simulink model "STDiscovery2016a"  (R2017b)
settings: Solver=FixedStepAuto  StartTime=0.0  StopTime=10  FixedStep=Abtastzeit  RelTol=1e-3
PreLoadFcn:
  | waijung.modelPreload; % Required for working with Waijung Blockset. Do not remove.
model workspace (MAT data in the model file):
  Abtastzeit = 0.01
  Servo_IN_min = 0.894
  SimulationDutyCycle = 27
undefined symbols (not defined in the file): HSEOSC, Link, LQFP176, ST, STM32F417IG
libraries: stm32f4_io_lib x15, simulink x10, simulink_extras x8, stm32f4_adc_lib x7, powerlib_meascontrol x3, stm32f4_device_config_lib x1
(part 5 of 5)

== system STDiscovery2016a/Aktorik/Ansteuerung Servo/Logik  ==
  Fernbedienung Signal : Inport
  Eingriff_Fernbedienung : Inport  Port=2
  Jetson Signal : Inport  Port=3
  "(Einschaltverzögerung) Wartezeit Anhalten " : powerlib_meascontrol/Logic/On Delay  DelayType=On delay  delay=1  ic=1  Ts=0
      settings: SourceProductName=Simscape Power Systems
  Data Type Conversion : DataTypeConversion  OutDataTypeStr=double
  "Erst 1s aktuellen autonomen Lenkeinschlag halten, dann Fernbedienung übernehmen" : Switch  Criteria=u2 > Threshold
  Modus Auswahl : Switch  Criteria=u2 > Threshold
  Output Pin : Outport
  wires:
  Data Type Conversion/1 -> "Erst 1s aktuellen autonomen Lenkeinschlag halten, dann Fernbedienung übernehmen"/1  "manuell"
  Eingriff_Fernbedienung/1 -> "(Einschaltverzögerung) Wartezeit Anhalten "/1, Modus Auswahl/2
  Modus Auswahl/1 -> Output Pin/1  "Ausgang zum servo"
  "Erst 1s aktuellen autonomen Lenkeinschlag halten, dann Fernbedienung übernehmen"/1 -> Modus Auswahl/1  "manuell"
  Jetson Signal/1 -> Modus Auswahl/3, "Erst 1s aktuellen autonomen Lenkeinschlag halten, dann Fernbedienung übernehmen"/3  "autonom"
  "(Einschaltverzögerung) Wartezeit Anhalten "/1 -> "Erst 1s aktuellen autonomen Lenkeinschlag halten, dann Fernbedienung übernehmen"/2
  Fernbedienung Signal/1 -> Data Type Conversion/1

== system STDiscovery2016a/Aktorik/Ansteuerung Servo/Plausibilitäts Check ==
  In1 : Inport
  "Gib Mittelstellung aus, wenn mit Signal etwas nicht Stimmt" : Switch  Criteria=u2 > Threshold
  Logical Operator : Logic  AllPortsSameDT=off  OutDataTypeStr=boolean
  Mittelstellung : Constant  Value=0.001407
  Relational Operator : RelationalOperator  Operator=<  OutDataTypeStr=boolean  RndMeth=Nearest
  Relational Operator1 : RelationalOperator  Operator=>  OutDataTypeStr=boolean  RndMeth=Nearest
  "ok max " : Constant  Value=0.0021
  ok min : Constant  Value=0.0008
  Out1 : Outport
  wires:
  In1/1 -> Relational Operator1/1, Relational Operator/1, "Gib Mittelstellung aus, wenn mit Signal etwas nicht Stimmt"/1
  Logical Operator/1 -> "Gib Mittelstellung aus, wenn mit Signal etwas nicht Stimmt"/2
  "Gib Mittelstellung aus, wenn mit Signal etwas nicht Stimmt"/1 -> Out1/1
  Mittelstellung/1 -> "Gib Mittelstellung aus, wenn mit Signal etwas nicht Stimmt"/3
  Relational Operator1/1 -> Logical Operator/2
  Relational Operator/1 -> Logical Operator/1
  ok min/1 -> Relational Operator1/2
  "ok max "/1 -> Relational Operator/2

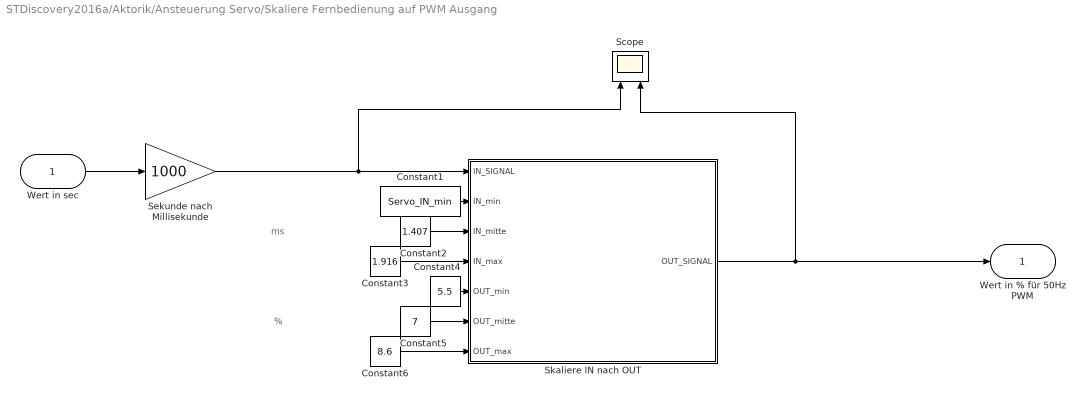
== system STDiscovery2016a/Aktorik/Ansteuerung Servo/Skaliere Fernbedienung auf PWM Ausgang ==
  note: %
  note: ms
  Wert in sec : Inport
  Constant1 : Constant  Value=Servo_IN_min
  Constant2 : Constant  Value=1.407
  Constant3 : Constant  Value=1.916
  Constant4 : Constant  Value=5.5
  Constant5 : Constant  Value=7
  Constant6 : Constant  Value=8.6
  Scope : Scope  NumInputPorts=2
  Sekunde nach Millisekunde : Gain  Gain=1000
  Skaliere lN nach OUT : Subsystem
  Wert in % für 50Hz PWM : Outport
  wires:
  Constant4/1 -> Skaliere lN nach OUT/5(OUT_min)
  Wert in sec/1 -> Sekunde nach Millisekunde/1
  Constant5/1 -> Skaliere lN nach OUT/6(OUT_mitte)
  Skaliere lN nach OUT/1(OUT_SIGNAL) -> Scope/2, Wert in % für 50Hz PWM/1
  Constant3/1 -> Skaliere lN nach OUT/4(IN_max)
  Constant2/1 -> Skaliere lN nach OUT/3(IN_mitte)
  Constant1/1 -> Skaliere lN nach OUT/2(IN_min)
  Constant6/1 -> Skaliere lN nach OUT/7(OUT_max)
  Sekunde nach Millisekunde/1 -> Scope/1, Skaliere lN nach OUT/1(IN_SIGNAL)

== system STDiscovery2016a/Aktorik/Ansteuerung Servo/Skaliere Stellwinkel auf PWM Ausgang ==
  note: %
  note: Stellwinkel
  Stellwinkel : Inport
  Constant1 : Constant  Value=-27
  Constant2 : Constant  Value=0
  Constant3 : Constant  Value=27
  Constant4 : Constant  Value=5.5
  Constant5 : Constant  Value=7
  Constant6 : Constant  Value=8.6
  Skaliere lN nach OUT : Subsystem
  Wert in % für 50Hz PWM : Outport
  wires:
  Constant4/1 -> Skaliere lN nach OUT/5(OUT_min)
  Constant5/1 -> Skaliere lN nach OUT/6(OUT_mitte)
  Skaliere lN nach OUT/1(OUT_SIGNAL) -> Wert in % für 50Hz PWM/1
  Constant3/1 -> Skaliere lN nach OUT/4(IN_max)
  Constant2/1 -> Skaliere lN nach OUT/3(IN_mitte)
  Constant1/1 -> Skaliere lN nach OUT/2(IN_min)
  Constant6/1 -> Skaliere lN nach OUT/7(OUT_max)
  Stellwinkel/1 -> Skaliere lN nach OUT/1(IN_SIGNAL)

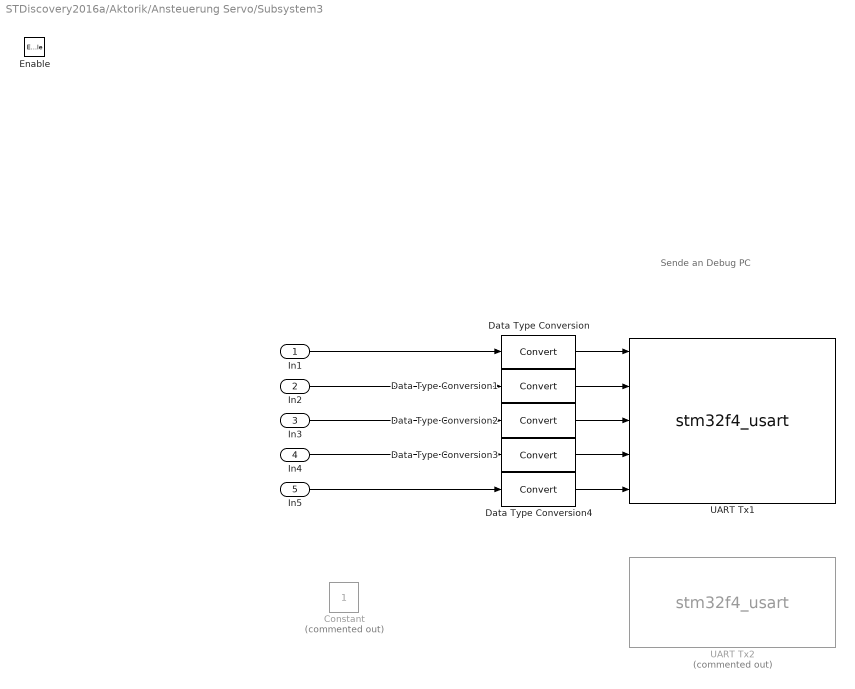
== system STDiscovery2016a/Aktorik/Ansteuerung Servo/Subsystem3 ==
  note: Sende an Debug PC
  In1 : Inport
  In2 : Inport  Port=2
  In3 : Inport  Port=3
  In4 : Inport  Port=4
  In5 : Inport  Port=5
  Enable : EnablePort
  Constant : Constant  Commented=on
  Data Type Conversion{,1..4} (5 alike) : DataTypeConversion
  UART Tx1 : S-Function  Priority=1  FunctionName=stm32f4_usart  Parameters=configuration,uartmodule,transfer,baudrate,inputtype,outputtype,confstr,binheaderarray,binterminatorarray,asciiheader,asciiterminator,bindatalength,packetmode,varname,sampletime,sampletimestr,blockid  SFunctionDeploymentMode=off  EnableBusSupport=off  mask(stm32f4_usart){configuration=Tx, uartmodule=3, baudrate=115200, databits=8, parity=No, stopbit=1, remaptxpin=Not used, remaprxpin=Not used, flowcontrol=None, remapctspin=Not used, remaprtspin=Not used, advanceoptions=off, rxbuffersize=512, txbuffersize=512, transfer=Blocking, packetmode=Ascii, binheader='7E 7E', binterminator='03 03', porttype_double=1, porttype_single=0, porttype_int8=1, porttype_uint8=0, porttype_int16=0, porttype_uint16=0, porttype_int32=0, porttype_uint32=0, asciiformat=' X: %f   ,Y:  %f , Lookahead: %f  , Geschwindigkeit: %f   ,Steuerbits(32):  %f', rx_asciiterminator=CRLF (0x0D 0x0A - "\r\n"), tx_asciiterminator=CRLF (0x0D 0x0A - "\r\n"), storagename=S, varname=, inputtype=[5  1 1 1 1 1], outputtype=[0], binheaderarray=[0], binterminatorarray=[0], bindatalength=0, asciiheader=' X: %f   ,Y:  %f , Lookahead: %f  , Geschwindigkeit: %f   ,Steuerbits(32):  %f\r\n', asciiterminator=[2 13 10], sampletime=0.1, sampletimestr=0.1, blockid=AktorikAnsteuerungServoSubsystem3UARTTx1, confstr=[ "dummy", "0", "*", "*", "0", "*", "*", "0", "*", "*", "0", "*", "*", "1", "4", "3", "1", "4", "1", "512", "512", "1", "3", "115200", "8", "No", "1", "None", "USART3"], lastmodule=1}
      mask prompts: uartmodule "UART Module"; baudrate "Baud rate (bps)"; databits "Data bits"; stopbit "Stop bit"; remaptxpin "Tx Pin"; remaprxpin "Rx Pin"; flowcontrol "Hardware flow control"; remapctspin "HW Flow control, CTS Pin"; remaprtspin "HW Flow control, RTS Pin"; advanceoptions "Advance options"; rxbuffersize "Rx buffer size (bytes)"; txbuffersize "Tx buffer size (bytes)"; packetmode "Packet mode"; binheader "Binary header (example: '7E 7E')"; binterminator "Binary terminator (example: '03 03')"; porttype_double "Number of data port, type DOUBLE"; porttype_single "Number of data port, type SINGLE"; porttype_int8 "Number of data port, type INT8"; porttype_uint8 "Number of data port, type UINT8"; porttype_int16 "Number of data port, type INT16"; porttype_uint16 "Number of data port, type UINT16"; porttype_int32 "Number of data port, type INT32"; porttype_uint32 "Number of data port, type UINT32"; asciiformat "Ascii format"; rx_asciiterminator "End of packet"; tx_asciiterminator "End of packet"; storagename "Buffer"; varname "Var name"; inputtype "Input data type"; outputtype "Output data type"; binheaderarray "Binary header"; binterminatorarray "Binary terminator"; bindatalength "Binary data length"; asciiheader "Ascii header (printf format)"; asciiterminator "Ascii terminator"; sampletime "Sample time (sec)"; sampletimestr "Compiled sample time (sec) in string"; confstr "Configuration string"; lastmodule "Last module selected"
      mask help:
      | Data type for Ascii format
      | %u, %i, %d, %o, %x: uint32
      | %e, %g, %f: single
      | %c: int8
      mask init:
      | stm32f4_usart_callback('init');
      mask Help: web(fullfile(waijungdocroot,'stm32f4_usart_tx.htm'), '-browser')
      mask TypeOptions configuration: Setup | Tx | Rx
      mask Callback configuration: stm32f4_usart_callback('configuration');
      mask TypeOptions uartmodule: 1 | 2 | 3 | 4 | 5 | 6
      mask Callback uartmodule: stm32f4_usart_callback('uartmodule');
      mask Callback baudrate: stm32f4_usart_callback('baudrate');
      mask TypeOptions databits: 8
      mask TypeOptions parity: No | Odd | Even
      mask TypeOptions stopbit: 0.5 | 1 | 1.5 | 2
      mask TypeOptions remaptxpin: Not used | A9 | B6
      mask TypeOptions remaprxpin: Not used | A10 | B7
      mask TypeOptions flowcontrol: None | RTS | CTS | RTS/CTS
      mask Callback flowcontrol: stm32f4_usart_callback('flowcontrol');
      mask TypeOptions remapctspin: Not used | A11
      mask TypeOptions remaprtspin: Not used | A12
      mask Callback advanceoptions: stm32f4_usart_callback('advanceoptions');
      mask TypeOptions rxbuffersize: 16 | 32 | 64 | 128 | 256 | 512 | 1024 | 2048
      mask TypeOptions txbuffersize: 16 | 32 | 64 | 128 | 256 | 512 | 1024 | 2048
      mask TypeOptions transfer: Blocking | Non-Blocking
      mask Callback transfer: stm32f4_usart_callback('transfer');
      mask TypeOptions packetmode: Ascii | Binary | String Buffer
      mask Callback packetmode: stm32f4_usart_callback('packetmode');
      mask Callback binheader: stm32f4_usart_callback('binheader');
      mask Callback binterminator: stm32f4_usart_callback('binterminator');
      mask Callback porttype_double: stm32f4_usart_callback('porttype');
      mask Callback porttype_single: stm32f4_usart_callback('porttype');
      mask Callback porttype_int8: stm32f4_usart_callback('porttype');
      mask Callback porttype_uint8: stm32f4_usart_callback('porttype');
      mask Callback porttype_int16: stm32f4_usart_callback('porttype');
      mask Callback porttype_uint16: stm32f4_usart_callback('porttype');
      mask Callback porttype_int32: stm32f4_usart_callback('porttype');
      mask Callback porttype_uint32: stm32f4_usart_callback('porttype');
      mask Callback asciiformat: stm32f4_usart_callback('asciiformat');
      mask TypeOptions rx_asciiterminator: CR (0x0D - "\r") | LF (0x0A - "\n") | CRLF (0x0D 0x0A - "\r\n")
      mask Callback rx_asciiterminator: stm32f4_usart_callback('rx_asciiterminator');
      mask TypeOptions tx_asciiterminator: CR (0x0D - "\r") | LF (0x0A - "\n") | CRLF (0x0D 0x0A - "\r\n") | None
      mask Callback tx_asciiterminator: stm32f4_usart_callback('tx_asciiterminator');
      mask TypeOptions storagename: <Please insert a storage name> | S
      mask Callback storagename: stm32f4_usart_callback('storagename');
      mask Callback varname: stm32f4_usart_callback('varname');
      mask Callback sampletime: stm32f4_usart_callback('sampletime');
      mask Callback sampletimestr: stm32f4_usart_callback('sampletimestr');
      mask Callback blockid: stm32f4_usart_callback('blockid');
      mask Display: text(0.95, 0.5, 'Module: USART3_Tx\nPacket: Ascii\nTransfer: Blocking\nTs (sec): 0.1','ver','middle','hor','right'); port_label('input', 1,'single'); port_label('input', 2,'single'); port_label('input', 3,'single'); port_label('input', 4,'single'); port_label('input', 5,'single');
  UART Tx2 : S-Function  Priority=1  Commented=on  FunctionName=stm32f4_usart  Parameters=configuration,uartmodule,transfer,baudrate,inputtype,outputtype,confstr,binheaderarray,binterminatorarray,asciiheader,asciiterminator,bindatalength,packetmode,varname,sampletime,sampletimestr,blockid  SFunctionDeploymentMode=off  EnableBusSupport=off  mask(stm32f4_usart){configuration=Tx, uartmodule=1, baudrate=115200, databits=8, parity=No, stopbit=1, remaptxpin=Not used, remaprxpin=Not used, flowcontrol=None, remapctspin=Not used, remaprtspin=Not used, advanceoptions=off, rxbuffersize=512, txbuffersize=512, transfer=Blocking, packetmode=Binary, binheader='', binterminator='', porttype_double=0, porttype_single=1, porttype_int8=0, porttype_uint8=0, porttype_int16=0, porttype_uint16=0, porttype_int32=0, porttype_uint32=0, asciiformat='Lookahead: %f   , X: %f   ,Y:  %f  ,Steuerbits(32):  %f', rx_asciiterminator=CRLF (0x0D 0x0A - "\r\n"), tx_asciiterminator=CRLF (0x0D 0x0A - "\r\n"), storagename=S, varname=, inputtype=[1  1], outputtype=[0], binheaderarray=[0 ], binterminatorarray=[0 ], bindatalength=4, asciiheader='Lookahead: %f   , X: %f   ,Y:  %f  ,Steuerbits(32):  %f\r\n', asciiterminator=[2 13 10], sampletime=0.1, sampletimestr=-1, blockid=AktorikAnsteuerungServoSubsystem3UARTTx2, confstr=[ "dummy", "0", "*", "*", "0", "*", "*", "0", "*", "*", "0", "*", "*", "2", "4", "7", "2", "4", "2", "512", "512", "2", "1", "115200", "8", "No", "1", "None", "USART1"], lastmodule=1}
      mask prompts: uartmodule "UART Module"; baudrate "Baud rate (bps)"; databits "Data bits"; stopbit "Stop bit"; remaptxpin "Tx Pin"; remaprxpin "Rx Pin"; flowcontrol "Hardware flow control"; remapctspin "HW Flow control, CTS Pin"; remaprtspin "HW Flow control, RTS Pin"; advanceoptions "Advance options"; rxbuffersize "Rx buffer size (bytes)"; txbuffersize "Tx buffer size (bytes)"; packetmode "Packet mode"; binheader "Binary header (example: '7E 7E')"; binterminator "Binary terminator (example: '03 03')"; porttype_double "Number of data port, type DOUBLE"; porttype_single "Number of data port, type SINGLE"; porttype_int8 "Number of data port, type INT8"; porttype_uint8 "Number of data port, type UINT8"; porttype_int16 "Number of data port, type INT16"; porttype_uint16 "Number of data port, type UINT16"; porttype_int32 "Number of data port, type INT32"; porttype_uint32 "Number of data port, type UINT32"; asciiformat "Ascii format"; rx_asciiterminator "End of packet"; tx_asciiterminator "End of packet"; storagename "Buffer"; varname "Var name"; inputtype "Input data type"; outputtype "Output data type"; binheaderarray "Binary header"; binterminatorarray "Binary terminator"; bindatalength "Binary data length"; asciiheader "Ascii header (printf format)"; asciiterminator "Ascii terminator"; sampletime "Sample time (sec)"; sampletimestr "Compiled sample time (sec) in string"; confstr "Configuration string"; lastmodule "Last module selected"
      mask help:
      | Data type for Ascii format
      | %u, %i, %d, %o, %x: uint32
      | %e, %g, %f: single
      | %c: int8
      mask init:
      | stm32f4_usart_callback('init');
      mask Help: web(fullfile(waijungdocroot,'stm32f4_usart_tx.htm'), '-browser')
      mask TypeOptions configuration: Setup | Tx | Rx
      mask Callback configuration: stm32f4_usart_callback('configuration');
      mask TypeOptions uartmodule: 1 | 2 | 3 | 4 | 5 | 6
      mask Callback uartmodule: stm32f4_usart_callback('uartmodule');
      mask Callback baudrate: stm32f4_usart_callback('baudrate');
      mask TypeOptions databits: 8
      mask TypeOptions parity: No | Odd | Even
      mask TypeOptions stopbit: 0.5 | 1 | 1.5 | 2
      mask TypeOptions remaptxpin: Not used | A9 | B6
      mask TypeOptions remaprxpin: Not used | A10 | B7
      mask TypeOptions flowcontrol: None | RTS | CTS | RTS/CTS
      mask Callback flowcontrol: stm32f4_usart_callback('flowcontrol');
      mask TypeOptions remapctspin: Not used | A11
      mask TypeOptions remaprtspin: Not used | A12
      mask Callback advanceoptions: stm32f4_usart_callback('advanceoptions');
      mask TypeOptions rxbuffersize: 16 | 32 | 64 | 128 | 256 | 512 | 1024 | 2048
      mask TypeOptions txbuffersize: 16 | 32 | 64 | 128 | 256 | 512 | 1024 | 2048
      mask TypeOptions transfer: Blocking | Non-Blocking
      mask Callback transfer: stm32f4_usart_callback('transfer');
      mask TypeOptions packetmode: Ascii | Binary | String Buffer
      mask Callback packetmode: stm32f4_usart_callback('packetmode');
      mask Callback binheader: stm32f4_usart_callback('binheader');
      mask Callback binterminator: stm32f4_usart_callback('binterminator');
      mask Callback porttype_double: stm32f4_usart_callback('porttype');
      mask Callback porttype_single: stm32f4_usart_callback('porttype');
      mask Callback porttype_int8: stm32f4_usart_callback('porttype');
      mask Callback porttype_uint8: stm32f4_usart_callback('porttype');
      mask Callback porttype_int16: stm32f4_usart_callback('porttype');
      mask Callback porttype_uint16: stm32f4_usart_callback('porttype');
      mask Callback porttype_int32: stm32f4_usart_callback('porttype');
      mask Callback porttype_uint32: stm32f4_usart_callback('porttype');
      mask Callback asciiformat: stm32f4_usart_callback('asciiformat');
      mask TypeOptions rx_asciiterminator: CR (0x0D - "\r") | LF (0x0A - "\n") | CRLF (0x0D 0x0A - "\r\n")
      mask Callback rx_asciiterminator: stm32f4_usart_callback('rx_asciiterminator');
      mask TypeOptions tx_asciiterminator: CR (0x0D - "\r") | LF (0x0A - "\n") | CRLF (0x0D 0x0A - "\r\n") | None
      mask Callback tx_asciiterminator: stm32f4_usart_callback('tx_asciiterminator');
      mask TypeOptions storagename: <Please insert a storage name> | S
      mask Callback storagename: stm32f4_usart_callback('storagename');
      mask Callback varname: stm32f4_usart_callback('varname');
      mask Callback sampletime: stm32f4_usart_callback('sampletime');
      mask Callback sampletimestr: stm32f4_usart_callback('sampletimestr');
      mask Callback blockid: stm32f4_usart_callback('blockid');
      mask Display: text(0.95, 0.5, 'Module: USART1_Tx\nPacket: Binary\nTransfer: Blocking\nTs (sec): -1','ver','middle','hor','right'); port_label('input', 1,'single');
  wires:
  In1/1 -> Data Type Conversion/1
  In2/1 -> Data Type Conversion1/1
  Data Type Conversion/1 -> UART Tx1/1
  Data Type Conversion2/1 -> UART Tx1/3
  Data Type Conversion1/1 -> UART Tx1/2
  In3/1 -> Data Type Conversion2/1
  In4/1 -> Data Type Conversion3/1
  Data Type Conversion3/1 -> UART Tx1/4
  In5/1 -> Data Type Conversion4/1
  Data Type Conversion4/1 -> UART Tx1/5

== system STDiscovery2016a/Aktorik/Ueberwachung ob Eingriff durch Fernbedienung/Motor Überwachung Eingriff durch Fernbedienung? ==
  Dutycycle in % : Inport
  Betrag bilden für negative Abweichunge : Abs
  Ist die Aktuelle Abweichung größer als die Maximal erlaubte? : RelationalOperator  Operator=>  OutDataTypeStr=boolean  RndMeth=Nearest
  Maximale Abweichung : Constant  Value=0.2
  "Mittelwert, in % wenn Fernsteuerung in der Mitte steht" : Constant  Value=7.45
  Subtract : Sum  Inputs=|+-
  Ja/Nein : Outport
  wires:
  "Mittelwert, in % wenn Fernsteuerung in der Mitte steht"/1 -> Subtract/2
  Betrag bilden für negative Abweichunge/1 -> Ist die Aktuelle Abweichung größer als die Maximal erlaubte?/1
  Maximale Abweichung/1 -> Ist die Aktuelle Abweichung größer als die Maximal erlaubte?/2
  Dutycycle in %/1 -> Subtract/1
  Subtract/1 -> Betrag bilden für negative Abweichunge/1
  Ist die Aktuelle Abweichung größer als die Maximal erlaubte?/1 -> Ja/Nein/1

== system STDiscovery2016a/Aktorik/Ueberwachung ob Eingriff durch Fernbedienung/Servo Überwachung Eingriff durch Fernbedienung? ==
  Dutycycle in % : Inport
  Betrag bilden für negative Abweichungen : Abs
  Ist die aktuelle Abweichung größer als die maximal erlaubte? : RelationalOperator  Operator=>  OutDataTypeStr=boolean  RndMeth=Nearest
  Maximale Abweichung : Constant  Value=0.2
  "Mittelwert, in % wenn Fernsteuerung in der Mitte steht" : Constant  Value=7
  Subtract : Sum  Inputs=|+-
  Ja/Nein : Outport
  wires:
  "Mittelwert, in % wenn Fernsteuerung in der Mitte steht"/1 -> Subtract/2
  Betrag bilden für negative Abweichungen/1 -> Ist die aktuelle Abweichung größer als die maximal erlaubte?/1
  Maximale Abweichung/1 -> Ist die aktuelle Abweichung größer als die maximal erlaubte?/2
  Dutycycle in %/1 -> Subtract/1
  Subtract/1 -> Betrag bilden für negative Abweichungen/1
  Ist die aktuelle Abweichung größer als die maximal erlaubte?/1 -> Ja/Nein/1

== system STDiscovery2016a/Debug/Subsystem/Safety 2.5 |<--->|12.5 ==
  In1 : Inport
  Constant : Constant  Value=2.5
  Constant1 : Constant  Value=12.5
  Data Type Conversion : DataTypeConversion
  Data Type Conversion1 : DataTypeConversion
  Switch : Switch  Criteria=u2 > Threshold  Threshold=2.5
  Switch1 : Switch  Criteria=u2 > Threshold  Threshold=12.5
  Out1 : Outport
  wires:
  Switch/1 -> Switch1/3, Switch1/2
  In1/1 -> Switch/1, Switch/2
  Switch1/1 -> Out1/1
  Constant/1 -> Data Type Conversion/1
  Constant1/1 -> Data Type Conversion1/1
  Data Type Conversion1/1 -> Switch1/1
  Data Type Conversion/1 -> Switch/3

== system STDiscovery2016a/Debug/Subsystem1/Safety 2.5 |<--->|12.5 ==
  In1 : Inport
  Constant : Constant  Value=2.5
  Constant1 : Constant  Value=12.5
  Data Type Conversion : DataTypeConversion
  Data Type Conversion1 : DataTypeConversion
  Switch : Switch  Criteria=u2 > Threshold  Threshold=2.5
  Switch1 : Switch  Criteria=u2 > Threshold  Threshold=12.5
  Out1 : Outport
  wires:
  Switch/1 -> Switch1/3, Switch1/2
  In1/1 -> Switch/1, Switch/2
  Switch1/1 -> Out1/1
  Constant/1 -> Data Type Conversion/1
  Constant1/1 -> Data Type Conversion1/1
  Data Type Conversion1/1 -> Switch1/1
  Data Type Conversion/1 -> Switch/3

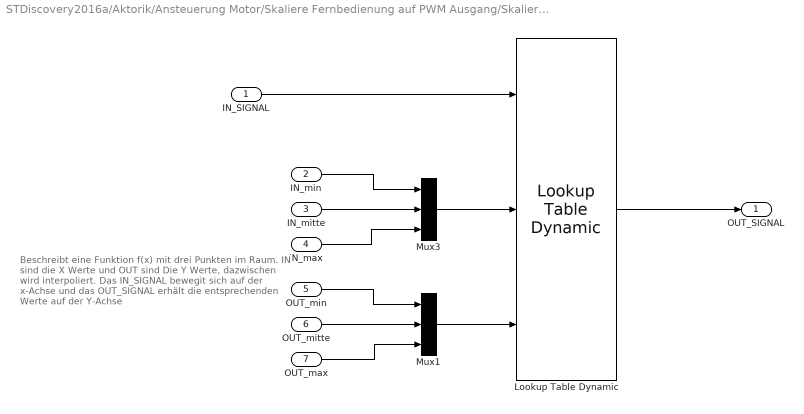
== system STDiscovery2016a/Aktorik/Ansteuerung Motor/Skaliere Fernbedienung auf PWM Ausgang/Skaliere lN nach OUT ==
  note: Beschreibt eine Funktion f(x) mit drei Punkten im Raum.
      | IN sind die X Werte und OUT sind Die Y Werte,
      | dazwischen wird interpoliert.
      |
      | Das IN_SIGNAL bewegit sich auf der x-Achse und
      | das OUT_SIGNAL erhält die entsprechenden Werte auf
      | der Y-Achse
  IN_SIGNAL : Inport
  IN_min : Inport  Port=2
  IN_mitte : Inport  Port=3
  IN_max : Inport  Port=4
  OUT_min : Inport  Port=5
  OUT_mitte : Inport  Port=6
  OUT_max : Inport  Port=7
  Lookup Table Dynamic : simulink/Lookup Tables/Lookup Table Dynamic  LookUpMeth=Interpolation-Use End Values  OutDataType=fixdt('double')  OutScaling=[]  OutputDataTypeScalingMode=Specify via dialog  OutDataTypeStr=fixdt('double')  DoSatur=off
      settings: SourceProductName=Simulink
  Mux1 : Mux  Inputs=3
  Mux3 : Mux  Inputs=3
  OUT_SIGNAL : Outport
  wires:
  IN_SIGNAL/1 -> Lookup Table Dynamic/1
  IN_max/1 -> Mux3/3
  IN_mitte/1 -> Mux3/2
  IN_min/1 -> Mux3/1
  OUT_min/1 -> Mux1/1
  OUT_mitte/1 -> Mux1/2
  OUT_max/1 -> Mux1/3
  Lookup Table Dynamic/1 -> OUT_SIGNAL/1
  Mux1/1 -> Lookup Table Dynamic/3
  Mux3/1 -> Lookup Table Dynamic/2

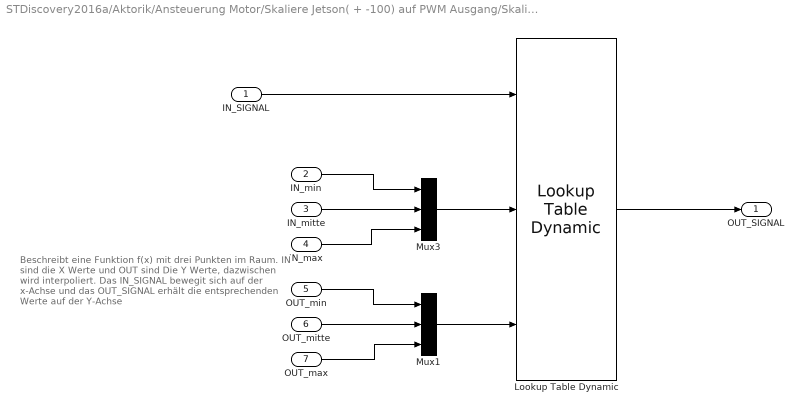
== system STDiscovery2016a/Aktorik/Ansteuerung Motor/Skaliere Jetson( + -100) auf PWM Ausgang/Skaliere lN nach OUT ==
  note: Beschreibt eine Funktion f(x) mit drei Punkten im Raum.
      | IN sind die X Werte und OUT sind Die Y Werte,
      | dazwischen wird interpoliert.
      |
      | Das IN_SIGNAL bewegit sich auf der x-Achse und
      | das OUT_SIGNAL erhält die entsprechenden Werte auf
      | der Y-Achse
  IN_SIGNAL : Inport
  IN_min : Inport  Port=2
  IN_mitte : Inport  Port=3
  IN_max : Inport  Port=4
  OUT_min : Inport  Port=5
  OUT_mitte : Inport  Port=6
  OUT_max : Inport  Port=7
  Lookup Table Dynamic : simulink/Lookup Tables/Lookup Table Dynamic  LookUpMeth=Interpolation-Use End Values  OutDataType=fixdt('double')  OutScaling=[]  OutputDataTypeScalingMode=Specify via dialog  OutDataTypeStr=fixdt('double')  DoSatur=off
      settings: SourceProductName=Simulink
  Mux1 : Mux  Inputs=3
  Mux3 : Mux  Inputs=3
  OUT_SIGNAL : Outport
  wires:
  IN_SIGNAL/1 -> Lookup Table Dynamic/1
  IN_max/1 -> Mux3/3
  IN_mitte/1 -> Mux3/2
  IN_min/1 -> Mux3/1
  OUT_min/1 -> Mux1/1
  OUT_mitte/1 -> Mux1/2
  OUT_max/1 -> Mux1/3
  Lookup Table Dynamic/1 -> OUT_SIGNAL/1
  Mux1/1 -> Lookup Table Dynamic/3
  Mux3/1 -> Lookup Table Dynamic/2

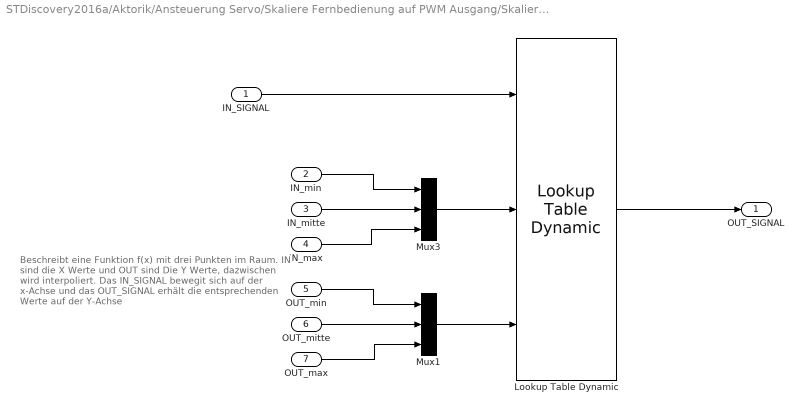
== system STDiscovery2016a/Aktorik/Ansteuerung Servo/Skaliere Fernbedienung auf PWM Ausgang/Skaliere lN nach OUT ==
  note: Beschreibt eine Funktion f(x) mit drei Punkten im Raum.
      | IN sind die X Werte und OUT sind Die Y Werte,
      | dazwischen wird interpoliert.
      |
      | Das IN_SIGNAL bewegit sich auf der x-Achse und
      | das OUT_SIGNAL erhält die entsprechenden Werte auf
      | der Y-Achse
  IN_SIGNAL : Inport
  IN_min : Inport  Port=2
  IN_mitte : Inport  Port=3
  IN_max : Inport  Port=4
  OUT_min : Inport  Port=5
  OUT_mitte : Inport  Port=6
  OUT_max : Inport  Port=7
  Lookup Table Dynamic : simulink/Lookup Tables/Lookup Table Dynamic  LookUpMeth=Interpolation-Use End Values  OutDataType=fixdt('double')  OutScaling=[]  OutputDataTypeScalingMode=Specify via dialog  OutDataTypeStr=fixdt('double')  DoSatur=off
      settings: SourceProductName=Simulink
  Mux1 : Mux  Inputs=3
  Mux3 : Mux  Inputs=3
  OUT_SIGNAL : Outport
  wires:
  IN_SIGNAL/1 -> Lookup Table Dynamic/1
  IN_max/1 -> Mux3/3
  IN_mitte/1 -> Mux3/2
  IN_min/1 -> Mux3/1
  OUT_min/1 -> Mux1/1
  OUT_mitte/1 -> Mux1/2
  OUT_max/1 -> Mux1/3
  Lookup Table Dynamic/1 -> OUT_SIGNAL/1
  Mux1/1 -> Lookup Table Dynamic/3
  Mux3/1 -> Lookup Table Dynamic/2

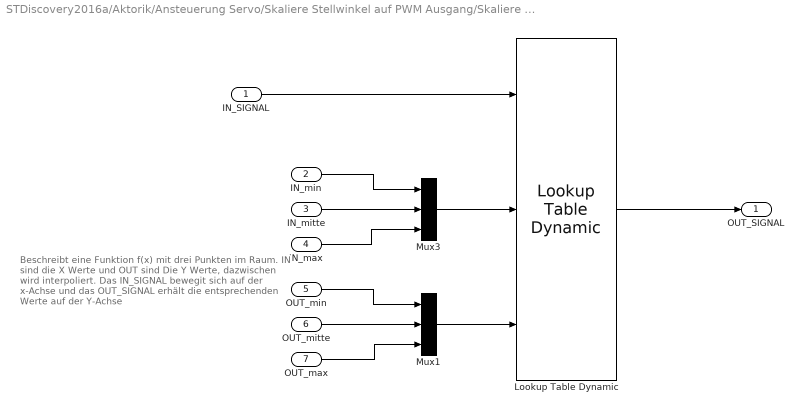
== system STDiscovery2016a/Aktorik/Ansteuerung Servo/Skaliere Stellwinkel auf PWM Ausgang/Skaliere lN nach OUT ==
  note: Beschreibt eine Funktion f(x) mit drei Punkten im Raum.
      | IN sind die X Werte und OUT sind Die Y Werte,
      | dazwischen wird interpoliert.
      |
      | Das IN_SIGNAL bewegit sich auf der x-Achse und
      | das OUT_SIGNAL erhält die entsprechenden Werte auf
      | der Y-Achse
  IN_SIGNAL : Inport
  IN_min : Inport  Port=2
  IN_mitte : Inport  Port=3
  IN_max : Inport  Port=4
  OUT_min : Inport  Port=5
  OUT_mitte : Inport  Port=6
  OUT_max : Inport  Port=7
  Lookup Table Dynamic : simulink/Lookup Tables/Lookup Table Dynamic  LookUpMeth=Interpolation-Use End Values  OutDataTypeStr=fixdt('double')  OutputDataTypeScalingMode=Specify via dialog  OutDataType=fixdt('double')  OutScaling=[]  DoSatur=off
      settings: SourceProductName=Simulink
  Mux1 : Mux  Inputs=3
  Mux3 : Mux  Inputs=3
  OUT_SIGNAL : Outport
  wires:
  IN_SIGNAL/1 -> Lookup Table Dynamic/1
  IN_max/1 -> Mux3/3
  IN_mitte/1 -> Mux3/2
  IN_min/1 -> Mux3/1
  OUT_min/1 -> Mux1/1
  OUT_mitte/1 -> Mux1/2
  OUT_max/1 -> Mux1/3
  Lookup Table Dynamic/1 -> OUT_SIGNAL/1
  Mux1/1 -> Lookup Table Dynamic/3
  Mux3/1 -> Lookup Table Dynamic/2

== matlab function STDiscovery2016a/Aktorik/Ansteuerung Servo/MATLAB Function ==
  data: Meter_Lookahead_Distance input; Phi_stell output; Meter_Yg input; v input; Phi_current input
function Phi_stell  = Path_Follower (Meter_Lookahead_Distance, Meter_Yg, v, Phi_current)



Radstand=0.27 %ToDo 27cm Radbreite: 15,7cm
c_ref=(2*Meter_Yg) / (Meter_Lookahead_Distance^2) %gewünschte Kurve
w_ref= v*c_ref %gewünschte Rotationsgeschwindigkeit
w_current= v*(tan(Phi_current)/Radstand) %momentane Rotationsgeschwindigkeit

e=w_ref-w_current %Abweichung aktuelle Winkelgeschwindigkeit zu gewünschter


Phi_stell=rad2deg(atan((e*Radstand)/v))
e=rad2deg(atan((e*Radstand)/v)) %Umrechnung Winkelgeschwindigkeit in stellwinkel
end
